simulink model "TrayectoriaStateFlow"  (R2023b)
settings: Solver=FixedStepAuto  StartTime=0.0  StopTime=50  RelTol=1e-3  EnableMultiTasking=on
model workspace (MAT data in the model file):
  d = 0.21
settings Model: ExtModeTrigDuration=2  Creator=Alberto  LastModifiedBy=Alberto
settings OptimizationCC: EnhancedBackFolding=on  PassReuseOutputArgsAs=Individual arguments  ZeroExternalMemoryAtStartup=off  ZeroInternalMemoryAtStartup=off  MaxStackSize=64  OptimizeBlockOrder=speed  DifferentSizesBufferReuse=on  OptimizationCustomize=off  EfficientTunableParamExpr=on
settings DebuggingCC: ParameterTunabilityLossMsg=error
settings HardwareCC: ProdBitPerInt=16  ProdBitPerPointer=16  ProdBitPerSizeT=16  ProdBitPerPtrDiffT=16  ProdLargestAtomicFloat=None  ProdWordSize=8  ProdHWDeviceType=Atmel->AVR  UseEmbeddedCoderFeatures=off  UseSimulinkCoderFeatures=off
settings SFSimCC: MATLABDynamicMemAlloc=off
settings RTWCC: Description=Embedded Coder  SystemTargetFile=ert.tlc  HardwareBoard=Arduino Mega 2560  TemplateMakefile=ert_default_tmf  Toolchain=Arduino AVR  BuildConfiguration=Faster Runs
settings CodeAppCC: ForceParamTrailComments=on  IgnoreCustomStorageClasses=off  OperatorAnnotations=on  SimulinkDataObjDesc=on  SFDataObjDesc=on  InsertBlockDesc=on
settings ERTTargetCC: SupportContinuousTime=on  SupportNonInlinedSFcns=on  SupportVariableSizeSignals=on  ExtModeTransport=3  ExtModeStaticAlloc=on  ExtModeAutomaticAllocSize=off  ExtModeStaticAllocSize=2048  ExtModeMexFile=ext_xcp  ExtModeIntrfLevel=Level2 - Open

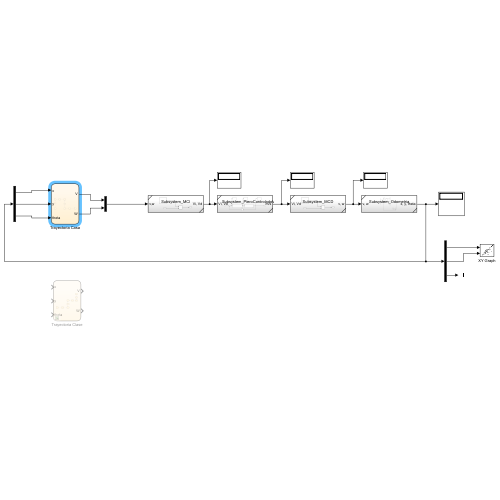
[thumbnail: Simulink's stored preview of the top-level diagram]
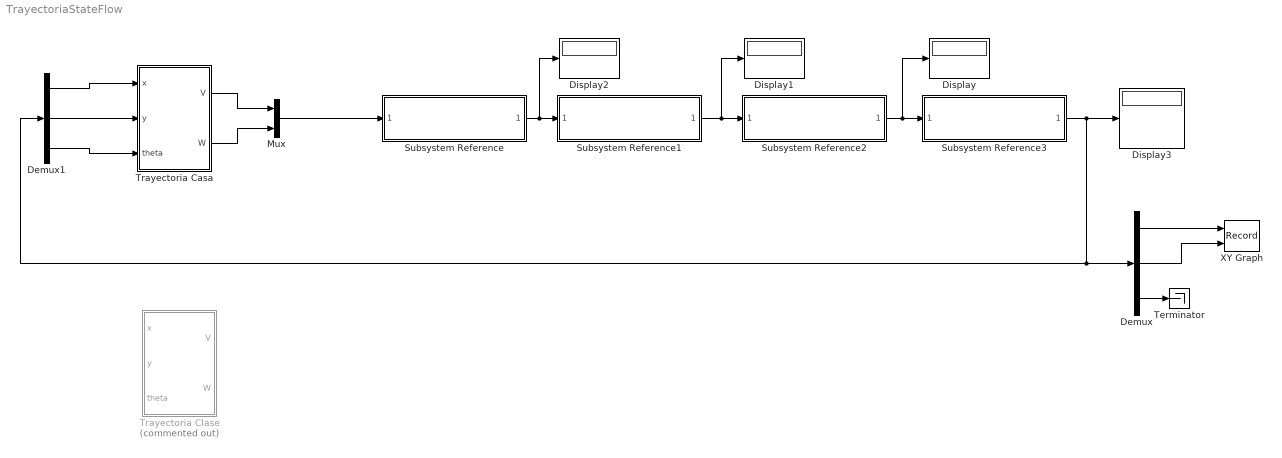
== system TrayectoriaStateFlow ==
  Demux : Demux  Outputs=3
  Demux1 : Demux  Outputs=3
  Display{,1..3} (4 alike) : Display
  Mux : Mux  Inputs=2
  Subsystem Reference : Subsystem  ReferencedSubsystem=Subsystem_MCI
  Subsystem Reference1 : Subsystem  ReferencedSubsystem=Subsystem_PieroControladoV
  Subsystem Reference2 : Subsystem  ReferencedSubsystem=Subsystem_MCD
  Subsystem Reference3 : Subsystem  ReferencedSubsystem=Subsystem_Odometria
  Terminator : Terminator
  Trayectoria Casa : Stateflow chart  TreatAsAtomicUnit=on
  Trayectoria Clase : Stateflow chart  Commented=on  TreatAsAtomicUnit=on
  XY Graph : Record  FileSettingsInternal="{\"entries\":[{\"content\":{\"excelSettings\":{\"content\":{},\"type\":\"Streamout.ExcelSettings\"}},\"type\":\"Streamout.FileSettingStorage\",\"uuid\":\"\"}],\"packageUris\":[\"http:\\/\\/schema.mathworks.com\\/mf0\\/streamout_blocks\\/R2020a\"],\"version\":\"1.0\"}"  Layout=[1 1]  SignalsInternal="{\"entries\":[{\"content\":{\"signals\":[{\"content\":{\"blockPath\":[],\"dimensions\":[1],\"domain\":\"\",\"lineColor\":\"#ff6929\",\"plots\":[ 1 ],\"port\":1,\"sid\":[\"\"],\"signalID\":1,\"signalName\":\"Demux:1\"},\"type\":\"RecordBlkView.Signal\",\"uuid\":\"\"},{\"content\":{\"blockPath\":[],\"dimensions\":[1],\"domain\":\"\",\"lineColor\":\"#b746ff\",\"plots\":[ 1 ],\"port\":2,\"sid\":[\"\"],\"signalID\":2,\"signalName\":\"Demux:2\"},\"type\":\"RecordBlkView.Signal\",\"uuid\":\"\"}]},\"type\":\"RecordBlkView.InputSignals\",\"uuid\":\"\"}],\"packageUris\":[\"http:\\/\\/schema.mathworks.com\\/mf0\\/streamout_blocks\\/R2020a\"],\"version\":\"1.0\"}"  VisualizationBindings="{\"xyplotplugin\":{\"info\":[{\"series\":[{\"bindingParametersList\":[{\"parameter\":\"X-Axis\",\"signalID\":1,\"signalName\":\"Demux:1\"},{\"parameter\":\"Y-Axis\",\"signalID\":2,\"signalName\":\"Demux:2\"}],\"seriesID\":0}],\"subplotID\":1}]}}"  CompatibilityTag=XY
  wires:
  Subsystem Reference2/1 -> Display/1, Subsystem Reference3/1
  Subsystem Reference1/1 -> Display1/1, Subsystem Reference2/1
  Subsystem Reference3/1 -> Demux1/1, Demux/1, Display3/1
  Mux/1 -> Subsystem Reference/1
  Subsystem Reference/1 -> Display2/1, Subsystem Reference1/1
  Trayectoria Casa/1(V) -> Mux/1
  Trayectoria Casa/2(W) -> Mux/2
  Demux1/1 -> Trayectoria Casa/1(x)
  Demux1/2 -> Trayectoria Casa/2(y)
  Demux1/3 -> Trayectoria Casa/3(theta)
  Demux/1 -> XY Graph/1
  Demux/2 -> XY Graph/2
  Demux/3 -> Terminator/1

== stateflow chart TrayectoriaStateFlow/Trayectoria Clase ==
  state Stop
    V=0;
    W=0;
  state GoStraight4m
    V=0.205;
    W=0;
  state rightTurn
    V=0.1;
    W=-pi/4;
  state GoStraight1m
    V=0.205;
    W=0;
  state LeftTurn1
    V=0.1;
    W=pi/4;
  state GoStraight12m
    V=0.205;
    W=0;
  state Inicio
    entry:
    V=0;
    W=0;
  state GoStraight
    V=0.205;
    W=0;
  state LeftTurn
    V=0.1;
    W=pi/4;
  GoStraight4m -> Stop : [y>14]
  LeftTurn1 -> GoStraight4m : [theta>pi/2]
  rightTurn -> GoStraight1m : [theta<0]
  GoStraight1m -> LeftTurn1 : [x>3]
  GoStraight12m -> rightTurn : [y>12]
  LeftTurn -> GoStraight12m : [theta>pi/2]
  (default) -> Inicio
  GoStraight -> LeftTurn : [x>2.1]
  Inicio -> GoStraight : [after (1, sec)]
  data: V output double size=1; W output double size=1; x input; y input; theta input

== stateflow chart TrayectoriaStateFlow/Trayectoria Casa ==
  state LeftTurn1
    V=0.1;
    W=pi/4;
  state GoStraight1m
    V=0.205;
    W=0;
  state LeftTurn
    V=0.1;
    W=pi/4;
  state GoStraigh2m
    V=0.205;
    W=0;
  state GoStraight4m
    V=0.205;
    W=0;
  state Stop
    V=0;
    W=0;
  state RightTurn
    V=0.1;
    W=-pi/4;
  state GoStraight
    V=0.205;
    W=0;
  state Inicio
    entry:
    V=0;
    W=0;
  GoStraight1m -> LeftTurn1 : [x>2.5]
  LeftTurn -> GoStraight1m : [theta>0-0.2]
  LeftTurn1 -> GoStraigh2m : [theta>pi/2-0.2]
  GoStraight4m -> LeftTurn : [y<-4.5]
  GoStraigh2m -> Stop : [y>-3]
  RightTurn -> GoStraight4m : [theta<-pi/2+0.2]
  (default) -> Inicio
  GoStraight -> RightTurn : [x>0.8]
  Inicio -> GoStraight : [after (1, sec)]
  data: V output double size=1; W output double size=1; x input; y input; theta input
